simulink model "transmit_LSF"  (R2024b)
settings: Solver=FixedStepAuto  StartTime=0.0  StopTime=0  FixedStep=1  RelTol=1e-3
values from neighbouring files (symbols this model uses):
  RandomizeSequence = hexToArray(RandomizeSequence,0)    [Full_transmit.m]
  SBLSF = hexToArray(SBLSF,1)    [Full_transmit.m]
libraries: simulink x2, commcnvcod2 x1, commblkintrlv2 x1
settings Model: Creator=fredr  LastModifiedBy=fredr

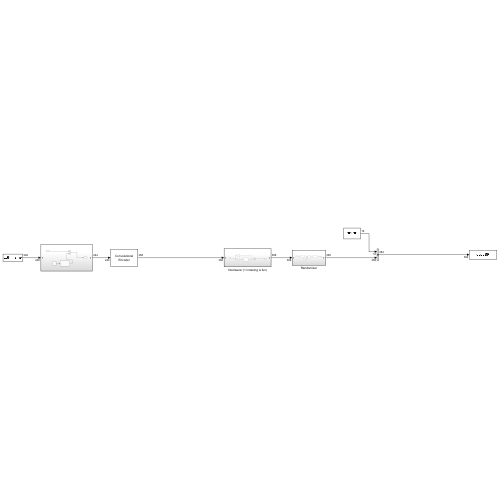
[thumbnail: Simulink's stored preview of the top-level diagram]
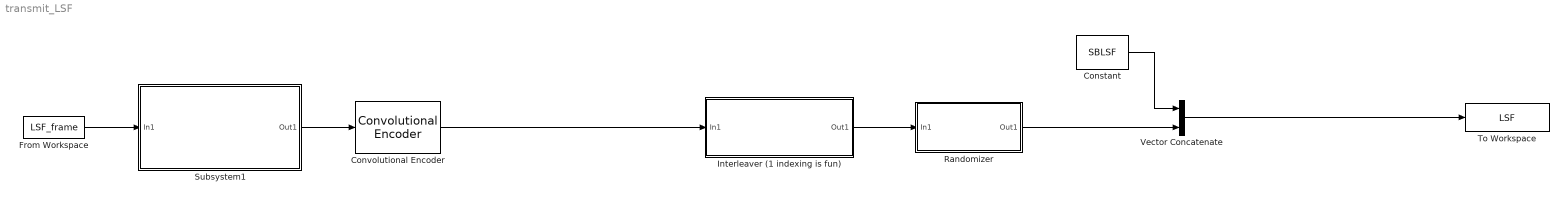
== system transmit_LSF ==
  Constant : Constant  Value=SBLSF
  Convolutional Encoder : commcnvcod2/Convolutional Encoder  trellis=poly2trellis(5, [23 35])  opMode=Continuous  DelayedResetAction=on  hasIniStPort=off  hasFinStPort=off  usePuncVector=on  punctureVector=P1  reset=Unused parameter value
      settings: LibrarySourceBlock=|
      | commhdlcnvcod/Convolutional
      | Encoder
  From Workspace : FromWorkspace  VariableName=LSF_frame
  Interleaver (1 indexing is fun) : Subsystem
  Randomizer : Subsystem
  Subsystem1 : Subsystem
  To Workspace : ToWorkspace  VariableName=LSF  SampleTime=-1
      settings: Save2DSignal=2-D array (concatenate along first dimension)
  Vector Concatenate : Concatenate
  wires:
  Randomizer/1(Out1) -> Vector Concatenate/2
  Vector Concatenate/1 -> To Workspace/1
  Constant/1 -> Vector Concatenate/1
  Interleaver (1 indexing is fun)/1(Out1) -> Randomizer/1(In1)
  Convolutional Encoder/1 -> Interleaver (1 indexing is fun)/1(In1)
  From Workspace/1 -> Subsystem1/1(In1)
  Subsystem1/1(Out1) -> Convolutional Encoder/1

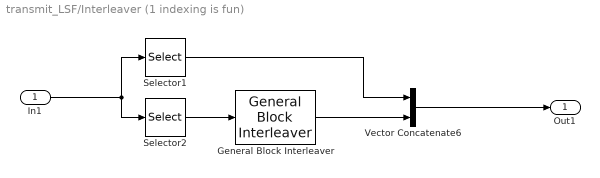
== system transmit_LSF/Interleaver (1 indexing is fun) ==
  In1 : Inport
  General Block Interleaver : commblkintrlv2/General Block Interleaver  StatePerturbationForJacobian=1.0e-05  permutationVectorSource=Dialog  elements=InterleavingVector
  Selector1 : Selector  IndexOptions=Index vector (dialog)  Indices=[1]  OutputSizes=1
  Selector2 : Selector  IndexOptions=Index vector (dialog)  Indices=[2:368]  OutputSizes=1
  Vector Concatenate6 : Concatenate
  Out1 : Outport
  wires:
  General Block Interleaver/1 -> Vector Concatenate6/2
  Selector1/1 -> Vector Concatenate6/1
  In1/1 -> Selector2/1, Selector1/1
  Selector2/1 -> General Block Interleaver/1
  Vector Concatenate6/1 -> Out1/1

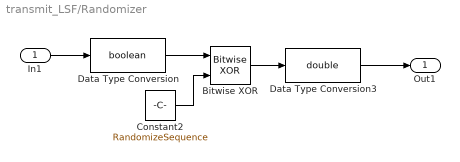
== system transmit_LSF/Randomizer ==
  In1 : Inport
  Bitwise XOR : simulink/Logic and Bit Operations/Bitwise Operator  logicop=XOR  UseBitMask=off  NumInputPorts=2  BitMask=bin2dec('11011001')  BitMaskRealWorld=Stored Integer
  Constant2 : Constant  Value=RandomizeSequence
  Data Type Conversion : DataTypeConversion  OutDataTypeStr=boolean  SaturateOnIntegerOverflow=off  RndMeth=Floor
  Data Type Conversion3 : DataTypeConversion  OutDataTypeStr=double  SaturateOnIntegerOverflow=off  RndMeth=Floor
  Out1 : Outport
  wires:
  Data Type Conversion/1 -> Bitwise XOR/1
  Data Type Conversion3/1 -> Out1/1
  In1/1 -> Data Type Conversion/1
  Constant2/1 -> Bitwise XOR/2
  Bitwise XOR/1 -> Data Type Conversion3/1

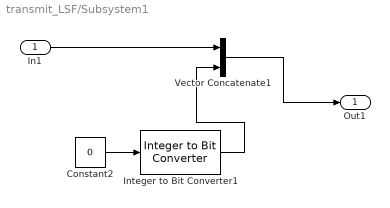
== system transmit_LSF/Subsystem1 ==
  In1 : Inport
  Constant2 : Constant  Value=0
  Integer to Bit Converter1 : simulink/Logic and Bit Operations/Integer to Bit Converter  nbits=4  signedInputValues=Unsigned  bitOrder=MSB first  outDtype=Inherit via internal rule
  Vector Concatenate1 : Concatenate
  Out1 : Outport
  wires:
  Vector Concatenate1/1 -> Out1/1
  Constant2/1 -> Integer to Bit Converter1/1
  Integer to Bit Converter1/1 -> Vector Concatenate1/2
  In1/1 -> Vector Concatenate1/1
